simulink model "SeatHeating"  (R2015a)
settings: Solver=FixedStepDiscrete  StartTime=0.0  StopTime=10.0  FixedStep=0.1  RelTol=1e-3
undefined symbols (not defined in the file): LeftHeatLevel, RightHeatLevel, SeatHeaterMain
settings Model: Creator=Morya  LastModifiedBy=Morya
settings DataIOCC: SaveFormat=StructureWithTime
settings OptimizationCC: ZeroExternalMemoryAtStartup=off  ZeroInternalMemoryAtStartup=off  OptimizeModelRefInitCode=on  LifeSpan=1
settings ModelReferenceCC: ModelReferenceNumInstancesAllowed=Single
settings RTWCC: SystemTargetFile=autosar.tlc  GenCodeOnly=on  TemplateMakefile=ert_default_tmf  Description=AUTOSAR
settings CodeAppCC: IgnoreCustomStorageClasses=off
settings STFCustomTargetCC: GenerateSampleERTMain=off  ParMdlRefBuildCompliant=on  CompOptLevelCompliant=on  IncludeMdlTerminateFcn=off  CombineOutputUpdateFcns=on  SuppressErrorStatus=on  ERTFirstTimeCompliant=on  SupportNonFinite=off  SupportComplex=off  SupportContinuousTime=off  SupportVariableSizeSignals=off  AutosarCompliant=on  SystemTargetFile=autosar.tlc
settings ERTTargetCC: GenerateSampleERTMain=off  ParMdlRefBuildCompliant=on  CompOptLevelCompliant=on  IncludeMdlTerminateFcn=off  SuppressErrorStatus=on  ERTFirstTimeCompliant=on  SupportNonFinite=off  SupportComplex=off  SupportContinuousTime=off  SupportVariableSizeSignals=off  AutosarCompliant=on  ERTCustomFileTemplate=example_file_process.tlc

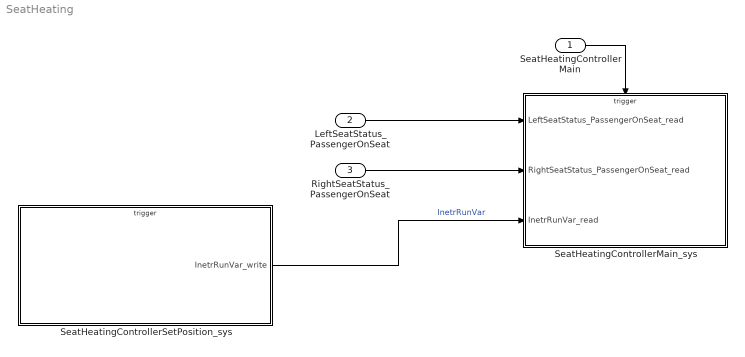
== system SeatHeating ==
  SeatHeatingControllerMain : Inport  OutputFunctionCall=on
  LeftSeatStatus_PassengerOnSeat : Inport  Port=2  OutDataTypeStr=boolean  PortDimensions=1
  RightSeatStatus_PassengerOnSeat : Inport  Port=3  OutDataTypeStr=boolean  PortDimensions=1
  SeatHeatingControllerMain_sys : Subsystem
  SeatHeatingControllerSetPosition_sys : Subsystem
  wires:
  SeatHeatingControllerMain/1 -> SeatHeatingControllerMain_sys/Trigger
  LeftSeatStatus_PassengerOnSeat/1 -> SeatHeatingControllerMain_sys/1(LeftSeatStatus_PassengerOnSeat_read)
  RightSeatStatus_PassengerOnSeat/1 -> SeatHeatingControllerMain_sys/2(RightSeatStatus_PassengerOnSeat_read)
  SeatHeatingControllerSetPosition_sys/1(InetrRunVar_write) -> SeatHeatingControllerMain_sys/3(InetrRunVar_read)  "InetrRunVar"

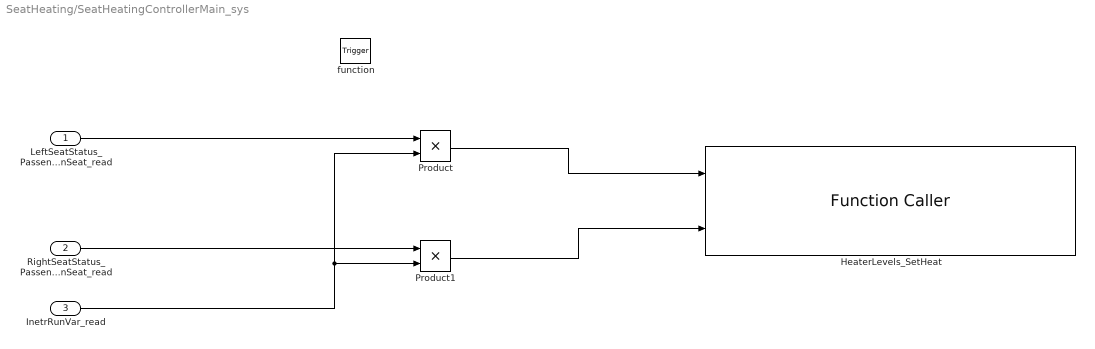
== system SeatHeating/SeatHeatingControllerMain_sys ==
  LeftSeatStatus_PassengerOnSeat_read : Inport
  RightSeatStatus_PassengerOnSeat_read : Inport  Port=2
  InetrRunVar_read : Inport  Port=3
  function : TriggerPort  TriggerType=function-call
  HeaterLevels_SetHeat : FunctionCaller  FunctionPrototype=SeatHeaterMain(LeftHeatLevel,RightHeatLevel)  InputArgumentSpecifications=P_Int32, P_Int32
  Product : Product  OutDataTypeStr=Inherit: Inherit via back propagation
  Product1 : Product  OutDataTypeStr=Inherit: Inherit via back propagation
  wires:
  RightSeatStatus_PassengerOnSeat_read/1 -> Product1/1
  InetrRunVar_read/1 -> Product1/2, Product/2
  LeftSeatStatus_PassengerOnSeat_read/1 -> Product/1
  Product1/1 -> HeaterLevels_SetHeat/2
  Product/1 -> HeaterLevels_SetHeat/1

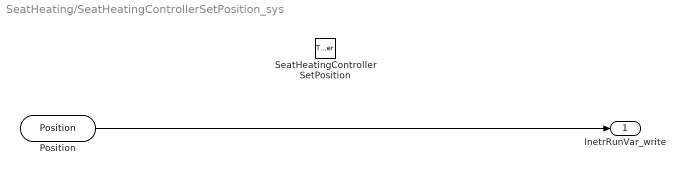
== system SeatHeating/SeatHeatingControllerSetPosition_sys ==
  SeatHeatingControllerSetPosition : TriggerPort  TriggerType=function-call  IsSimulinkFunction=on  FunctionName=SeatHeatingControllerSetPosition
  Position : ArgIn  OutDataTypeStr=Int32  ArgumentName=Position
  InetrRunVar_write : Outport  OutDataTypeStr=Int32  PortDimensions=1
  wires:
  Position/1 -> InetrRunVar_write/1
